simulink model "Simplified_Model"  (R2014a)
settings: Solver=ode45  StartTime=0.0  StopTime=10.0  RelTol=1e-3
settings Model: CovSFcnEnable=on  Creator=a_botros  LastModifiedBy=scorpii
settings OptimizationCC: SimCompilerOptimization=off
settings DebuggingCC: MergeDetectMultiDrivingBlocksExec=error  SolverPrmCheckMsg=none  FrameProcessingCompatibilityMsg=error
settings RTWCC: RTWCompilerOptimization=off

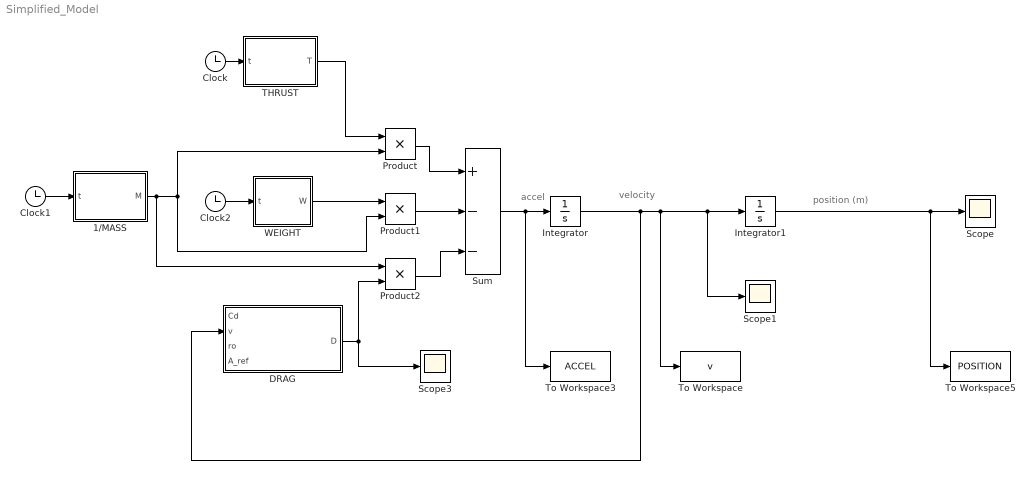
== system Simplified_Model ==
  note: position (m)
  note: velocity
  note: accel
  1/MASS : MATLAB Function  TreatAsAtomicUnit=on
  Clock : Clock
  Clock1 : Clock
  Clock2 : Clock
  DRAG : MATLAB Function  TreatAsAtomicUnit=on
  Integrator : Integrator
  Integrator1 : Integrator
  Product : Product
  Product1 : Product
  Product2 : Product
  Scope : Scope
  Scope1 : Scope
  Scope3 : Scope
      settings: SaveName=ScopeData3
  Sum : Sum  Inputs=+--
  THRUST : MATLAB Function  TreatAsAtomicUnit=on
  To Workspace : ToWorkspace  VariableName=v  SampleTime=-1
  To Workspace3 : ToWorkspace  VariableName=ACCEL  SaveFormat=Timeseries  SampleTime=-1
  To Workspace5 : ToWorkspace  VariableName=POSITION  SampleTime=-1
  WEIGHT : MATLAB Function  TreatAsAtomicUnit=on
  wires:
  THRUST/1(T) -> Product/1
  1/MASS/1(M) -> Product2/1, Product1/2, Product/2
  Clock/1 -> THRUST/1(t)
  Clock1/1 -> 1/MASS/1(t)
  Product/1 -> Sum/1
  Clock2/1 -> WEIGHT/1(t)
  Product1/1 -> Sum/2
  DRAG/1(D) -> Product2/2, Scope3/1
  Product2/1 -> Sum/3
  Integrator/1 -> DRAG/2(v), Scope1/1, Integrator1/1, To Workspace/1
  Sum/1 -> To Workspace3/1, Integrator/1
  WEIGHT/1(W) -> Product1/1
  Integrator1/1 -> To Workspace5/1, Scope/1

== matlab function Simplified_Model/WEIGHT ==
  data: t input; W output
function W   = WEIGHT( t )
if t<0.47775
    W=(-36625*t^4+32622*t^3-9361.4*t^2-112.87*t+21203)/1000*9.80665 
elseif t<4.0777
    W=(60.388*t^2-1213.3*t+21312)/1000*9.80665 
elseif t<4.5777
    W=(-144.73*t+18078)/1000*9.80665 
else
    W=17422/1000*9.80665 
end


end

== matlab function Simplified_Model/THRUST ==
  data: t input; T output
function  T  = THRUST(t)
%YIELDS THRUST CURVE OVER TIME
if t<0.08
    T=4000000*t^3-462933*t^2+41915*t+209.66
elseif t<0.15935
    T=-4701*t+2748.7
elseif t<0.21276 
    T=-1133.2*t+2223.6 
elseif t<0.32775
    T=787.15*t+1850.2
elseif t<0.57775
    T=-754.4*t+2339.9  
elseif t<0.72775
    T=-251*t+2070.7 
elseif t<1.7277
    T=-70.147*t+1947.4
elseif t<3.3777
    T=-31.421*t^2-9.1503*t+1930.8
elseif t<3.9777
    T=3656.6*t^3-39167*t^2+137806*t-158018
elseif t<4.5277
    T=-1051.8*t+4709.4
else
    T=0
    
      
   end


end

== matlab function Simplified_Model/1//MASS ==
  data: t input; M output
function M   = MASSRECIP( t )
if t<0.47775
    M=1/((-36625*t^4+32622*t^3-9361.4*t^2-112.87*t+21203)/1000)
elseif t<4.0777
    M=1/((60.388*t^2-1213.3*t+21312)/1000)
elseif t<4.5777
    M=1/((-144.73*t+18078)/1000)
else
    M=1/(17422/1000)
end


end

== matlab function Simplified_Model/DRAG ==
  data: Cd input; D output; v input; ro input; A_ref input
function D = DRAG(Cd, v, ro, A_ref)
%#codegen
D=0.5*Cd*v^2*A_ref*ro
end
